simulink model "p1a4"  (R2023b)
settings: Solver=VariableStepAuto  StartTime=0.0  StopTime=100.0  RelTol=1e-3
settings Model: Creator=tanvi  LastModifiedBy=tanvi

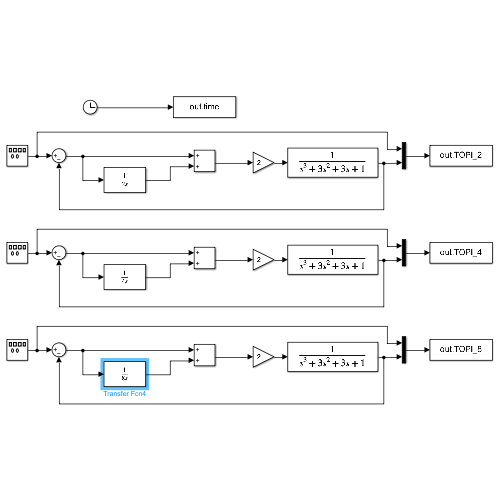
[thumbnail: Simulink's stored preview of the top-level diagram]
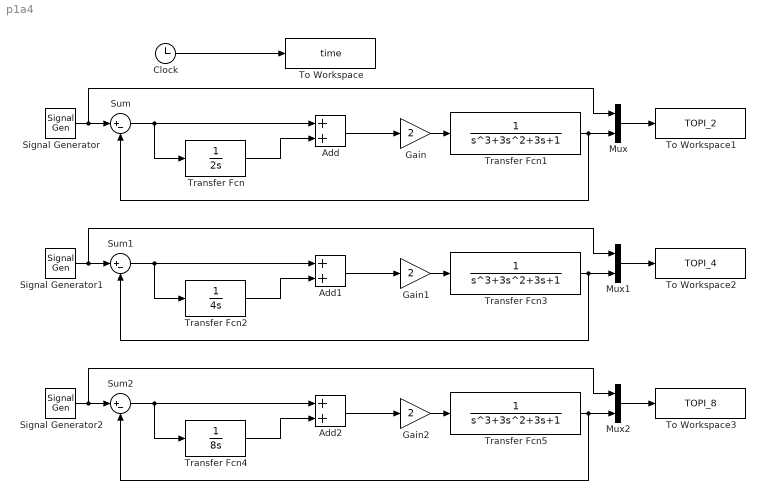
== system p1a4 ==
  Add : Sum
  Add1 : Sum
  Add2 : Sum
  Clock : Clock
  Gain : Gain  Gain=2
  Gain1 : Gain  Gain=2
  Gain2 : Gain  Gain=2
  Mux : Mux  Inputs=2
  Mux1 : Mux  Inputs=2
  Mux2 : Mux  Inputs=2
  Signal Generator : SignalGenerator  WaveForm=square  Frequency=0.01
  Signal Generator1 : SignalGenerator  WaveForm=square  Frequency=0.01
  Signal Generator2 : SignalGenerator  WaveForm=square  Frequency=0.01
  Sum : Sum  Inputs=|+-
  Sum1 : Sum  Inputs=|+-
  Sum2 : Sum  Inputs=|+-
  To Workspace : ToWorkspace  VariableName=time  SampleTime=-1
  To Workspace1 : ToWorkspace  VariableName=TOPI_2  SampleTime=-1
  To Workspace2 : ToWorkspace  VariableName=TOPI_4  SampleTime=-1
  To Workspace3 : ToWorkspace  VariableName=TOPI_8  SampleTime=-1
  Transfer Fcn : TransferFcn  Denominator=[2 0]
  Transfer Fcn1 : TransferFcn  Denominator=[1 3 3 1]
  Transfer Fcn2 : TransferFcn  Denominator=[4 0]
  Transfer Fcn3 : TransferFcn  Denominator=[1 3 3 1]
  Transfer Fcn4 : TransferFcn  Denominator=[8 0]
  Transfer Fcn5 : TransferFcn  Denominator=[1 3 3 1]
  wires:
  Signal Generator/1 -> Mux/1, Sum/1
  Sum/1 -> Transfer Fcn/1, Add/1
  Clock/1 -> To Workspace/1
  Transfer Fcn1/1 -> Sum/2, Mux/2
  Transfer Fcn/1 -> Add/2
  Mux/1 -> To Workspace1/1
  Add/1 -> Gain/1
  Gain/1 -> Transfer Fcn1/1
  Mux1/1 -> To Workspace2/1
  Transfer Fcn3/1 -> Sum1/2, Mux1/2
  Add1/1 -> Gain1/1
  Gain1/1 -> Transfer Fcn3/1
  Transfer Fcn2/1 -> Add1/2
  Signal Generator1/1 -> Mux1/1, Sum1/1
  Sum1/1 -> Transfer Fcn2/1, Add1/1
  Mux2/1 -> To Workspace3/1
  Transfer Fcn5/1 -> Sum2/2, Mux2/2
  Add2/1 -> Gain2/1
  Gain2/1 -> Transfer Fcn5/1
  Transfer Fcn4/1 -> Add2/2
  Signal Generator2/1 -> Mux2/1, Sum2/1
  Sum2/1 -> Transfer Fcn4/1, Add2/1
